simulink model "scattering_based_vel_vel"  (R2020b)
settings: Solver=ode45  StartTime=0.0  StopTime=10  RelTol=1e-3
values from neighbouring files (symbols this model uses):
  A = [1 Ts ... (first row only)    [kalman_hw6_main_vv.m]
  Amp = 0.8    [hw6_main_vv.m]    (also in kalman_hw6_main_vv.m = 0.3)
  b = 1    [hw6_main_vv.m]    (also in kalman_hw6_main_vv.m)
  Be = 20    [hw6_main_vv.m]    (also in kalman_hw6_main_vv.m)
  Bh = 1.5    [hw6_main_vv.m]    (also in kalman_hw6_main_vv.m)
  Bm = 10    [hw6_main_vv.m]    (also in kalman_hw6_main_vv.m)
  Bs = 100    [hw6_main_vv.m]    (also in kalman_hw6_main_vv.m)
  C = [1 0]    [kalman_hw6_main_vv.m]
  delay = 10    [hw6_main_vv.m]    (also in kalman_hw6_main_vv.m)
  Dh = 8    [hw6_main_vv.m]    (also in kalman_hw6_main_vv.m)
  Dm = 0    [hw6_main_vv.m]    (also in kalman_hw6_main_vv.m)
  Ds = 0    [hw6_main_vv.m]    (also in kalman_hw6_main_vv.m)
  Je = 0    [hw6_main_vv.m]    (also in kalman_hw6_main_vv.m)
  Jh = 0    [hw6_main_vv.m]    (also in kalman_hw6_main_vv.m)
  Ke = 210    [hw6_main_vv.m]    (also in kalman_hw6_main_vv.m)
  Kh = 0.1    [hw6_main_vv.m]    (also in kalman_hw6_main_vv.m)
  Km = 30    [hw6_main_vv.m]    (also in kalman_hw6_main_vv.m)
  Ks = 80    [hw6_main_vv.m]    (also in kalman_hw6_main_vv.m)
  Mm = 0.5    [hw6_main_vv.m]    (also in kalman_hw6_main_vv.m)
  Ms = 2    [hw6_main_vv.m]    (also in kalman_hw6_main_vv.m)
  Ph = 1    [hw6_main_vv.m]    (also in kalman_hw6_main_vv.m)
  posNoiseVar = 0.00001    (= 1e-05)    [kalman_hw6_main_vv.m]
  R_m = 1    [kalman_hw6_main_vv.m]
  R_s = 1    [kalman_hw6_main_vv.m]
  torqueNoiseVar = 0.01    [kalman_hw6_main_vv.m]
  Ts = 0.001    [hw6_main_vv.m]    (also in kalman_hw6_main_vv.m)
  xe = 0.5    [hw6_main_vv.m]    (also in kalman_hw6_main_vv.m)
undefined symbols (not defined in the file or in its folder): DiscIntNeverNeededParam, Discrete, Fc, Fip, Time
libraries: simulink x4, ctrlSharedLib x2
settings Model: Creator=nicol  LastModifiedBy=nicol

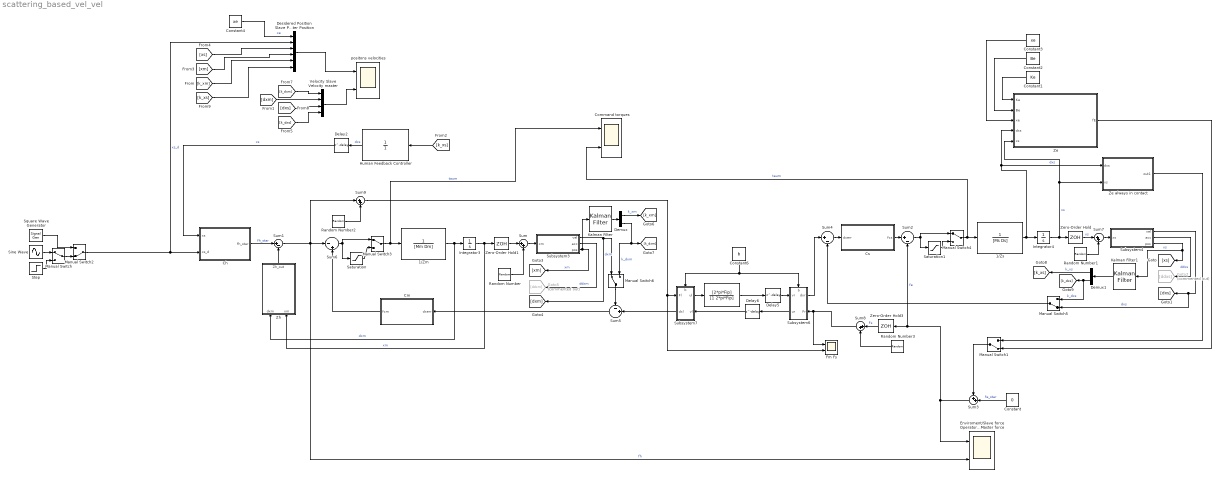
== system scattering_based_vel_vel ==
  " " : TransferFcn  Numerator=[2*pi*Fip]  Denominator=[1 2*pi*Fip]
  1/Zm : TransferFcn  Denominator=[Mm Dm]
  1/Zs : TransferFcn  Denominator=[Ms Ds]
  Ch : Subsystem
  Cm : Subsystem
  Command torques : Scope  NumInputPorts=2
  Constant : Constant  Value=0
  Constant1 : Constant  Value=Ke
  Constant2 : Constant  Value=Be
  Constant3 : Constant  Value=xe
  Constant4 : Constant  Value=xe
  Constant6 : Constant  Value=b
  Cs : Subsystem
  Delay2 : Delay  DelayLength=delay  SampleTime=Ts
  Delay5 : Delay  DelayLength=delay  SampleTime=Ts
  Delay6 : Delay  DelayLength=delay  SampleTime=Ts
  Demux : Demux  Outputs=2
  Demux1 : Demux  Outputs=2
  Desidered Position Slave Position Master Position : Mux  Inputs=6
  Enviroment/Slave force Operator/Master force : Scope  NumInputPorts=2
  Fm Fs : Scope  NumInputPorts=2
  Goto2 : Goto  Commented=on  GotoTag=ddxs
  Goto5 : Goto  Commented=on  GotoTag=ddxm
  Human Feedback Controller : TransferFcn  Denominator=[1]
  Integrator3 : Integrator
  Integrator4 : Integrator
  Kalman Filter : ctrlSharedLib/Kalman Filter  TimeDomain=Discrete-Time  UseCurrentEstimator=on  ModelSource=Individual A, B, C, D matrices  ModelSourceVariable=ss(0.95,1,0,0,Ts)  A=A  B=1  C=C  D=0  NumberOfStates=1  NumberOfInputs=1  NumberOfOutputs=1  InitialEstimateSource=Dialog  X0=0  P0=10  UseK=off  UseGH=off  NumberOfProcessNoiseInputs=1  G=1  TimeInvariantG=on  H=0  TimeInvariantH=on  Q=Q_m  TimeInvariantQ=on  R=R_m  TimeInvariantR=on  N=0  TimeInvariantN=on  AddInputPort=off  AddEnablePort=off  OutputEstimatedY=off  OutputP=off  Ts=Ts
  Kalman Filter1 : ctrlSharedLib/Kalman Filter  TimeDomain=Discrete-Time  UseCurrentEstimator=on  ModelSource=Individual A, B, C, D matrices  ModelSourceVariable=ss(0.95,1,0,0,Ts)  A=A  B=1  C=C  D=0  NumberOfStates=1  NumberOfInputs=1  NumberOfOutputs=1  InitialEstimateSource=Dialog  X0=0  P0=10  UseK=off  UseGH=off  NumberOfProcessNoiseInputs=1  G=1  TimeInvariantG=on  H=0  TimeInvariantH=on  Q=Q_s  TimeInvariantQ=on  R=R_s  TimeInvariantR=on  N=0  TimeInvariantN=on  AddInputPort=off  AddEnablePort=off  OutputEstimatedY=off  OutputP=off  Ts=Ts
  Manual Switch{,3..4,6} (4 alike) : ManualSwitch
  Manual Switch1 : ManualSwitch  CurrentSetting=0
  Manual Switch2 : ManualSwitch  CurrentSetting=0
  Manual Switch5 : ManualSwitch  CurrentSetting=0
  Random Number : RandomNumber  Variance=posNoiseVar  SampleTime=Ts
  Random Number1 : RandomNumber  Variance=posNoiseVar  SampleTime=Ts
  Random Number2 : RandomNumber  Variance=torqueNoiseVar  SampleTime=Ts
  Random Number3 : RandomNumber  Variance=torqueNoiseVar  SampleTime=Ts
  Saturation : Saturate  UpperLimit=50  LowerLimit=-50
  Saturation1 : Saturate  UpperLimit=50  LowerLimit=-50
  Sine Wave : Sin  Amplitude=Amp  Frequency=2*pi*Fc  SampleTime=0
  Square Wave Generator : SignalGenerator  WaveForm=square  Amplitude=Amp  Frequency=Fc  Units=rad/sec
  Step : Step  Time=Amp  SampleTime=0
  Subsystem3 : Subsystem
  Subsystem4 : Subsystem
  Subsystem6 : Subsystem
      settings: PortSchema="{\"entries\":[{\"content\":{\"sides\":[{\"content\":{\"connectorIds\":[\"In1\",\"Out2\"]},\"type\":\"ConnectorPlacement.EquallySpacedRectSide\",\"uuid\":\"6288401b-7cd3-4b91-bca2-5e472b2e7daa\"},{\"content\":{\"connectorIds\":[\"Out1\",\"In3\"],\"side\":\"RIGHT\"},\"type\":\"ConnectorPlacement.EquallySpacedRectSide\",\"uuid\":\"a26b0e98-9a48-48c5-be40-0718b6388037\"},{\"content\":{\"connectorIds\":[\"In2\"],\"side\":\"TOP\"},\"type\":\"ConnectorPlacement.EquallySpacedRectSide\",\"uuid\":\"663684a5-b6d6-4ce8-bd22-863e832b1e44\"},{\"content\":{\"connectorIds\":[],\"side\":\"HIDDEN\"},\"type\":\"ConnectorPlacement.EquallySpacedRectSide\",\"uuid\":\"305185ea-b8ab-4d44-85aa-b4ee32720aa4\"}]},\"type\":\"ConnectorPlacement.EquallySpacedConnector\",\"uuid\":\"5d1994be-23eb-41de-9d91-33fb6a380aab\"}],\"packageUris\":[\"http://schema.mathworks.com/mf0/Connector/R2020b\"],\"version\":\"1.0\"}"
  Subsystem7 : Subsystem
      settings: PortSchema="{\"entries\":[{\"content\":{\"sides\":[{\"content\":{\"connectorIds\":[\"In1\",\"Out2\"]},\"type\":\"ConnectorPlacement.EquallySpacedRectSide\",\"uuid\":\"6288401b-7cd3-4b91-bca2-5e472b2e7daa\"},{\"content\":{\"connectorIds\":[\"Out1\",\"In3\"],\"side\":\"RIGHT\"},\"type\":\"ConnectorPlacement.EquallySpacedRectSide\",\"uuid\":\"a26b0e98-9a48-48c5-be40-0718b6388037\"},{\"content\":{\"connectorIds\":[\"In2\"],\"side\":\"TOP\"},\"type\":\"ConnectorPlacement.EquallySpacedRectSide\",\"uuid\":\"663684a5-b6d6-4ce8-bd22-863e832b1e44\"},{\"content\":{\"connectorIds\":[],\"side\":\"HIDDEN\"},\"type\":\"ConnectorPlacement.EquallySpacedRectSide\",\"uuid\":\"305185ea-b8ab-4d44-85aa-b4ee32720aa4\"}]},\"type\":\"ConnectorPlacement.EquallySpacedConnector\",\"uuid\":\"5d1994be-23eb-41de-9d91-33fb6a380aab\"}],\"packageUris\":[\"http://schema.mathworks.com/mf0/Connector/R2020b\"],\"version\":\"1.0\"}"
  Sum{,7..9} (4 alike) : Sum  Inputs=|++
  Sum1 : Sum  Inputs=|+-
  Sum2 : Sum  Inputs=|+-
  Sum3 : Sum  Inputs=++|
  Sum4 : Sum  Inputs=|+-
  Sum5 : Sum  Inputs=-+|
  Sum6 : Sum  Inputs=|-+
  Velocity Slave Velocity master : Mux
  Ze : MATLAB Function  TreatAsAtomicUnit=on
  Ze always in contact : Subsystem
  Zero-Order Hold : ZeroOrderHold  SampleTime=Ts
  Zero-Order Hold1 : ZeroOrderHold  SampleTime=Ts
  Zero-Order Hold3 : ZeroOrderHold  SampleTime=Ts
  Zh : Subsystem
  "positons velocities " : Scope  NumInputPorts=2
  wires:
  Ch/1(fh_star) -> Sum1/1  "fh_star"
  Zh/1(Zh_out) -> Sum1/2
  1/Zm/1 -> Integrator3/1, Zh/1(dxm)  "dxm"
  Sum1/1 -> Sum9/1, Sum6/1, Enviroment/Slave force Operator/Master force/2  "fh"
  Cs/1(fcs) -> Sum2/1
  1/Zs/1 -> Integrator4/1, Ze always in contact/1(dxs), Ze/4(dxs)  "dxs"
  Ze/1(fE) -> Manual Switch1/2
  Sum3/1 -> Enviroment/Slave force Operator/Master force/1, Zero-Order Hold3/1, Sum2/2  "fe"
  Constant/1 -> Sum3/2  "fe_star"
  Constant1/1 -> Ze/1(Ke)
  Constant2/1 -> Ze/2(Be)
  Constant3/1 -> Ze/3(xe)
  Integrator4/1 -> Zero-Order Hold/1, Ze/5(xs), Ze always in contact/2(xs)  "xs"
  Sine Wave/1 -> Manual Switch/1
  Manual Switch1/1 -> Sum3/1
  Ze always in contact/1(out1) -> Manual Switch1/1
  Sum4/1 -> Cs/1(dxerr)
  Subsystem3/1(vel) -> Manual Switch6/1, [dxm]  "dxm"
  Subsystem3/3(pos) -> Kalman Filter/1, [xm]  "xm"
  Integrator3/1 -> Zero-Order Hold1/1, Zh/2(xm)  "xm"
  Subsystem3/2(acc) -> Goto5/1  "ddxm"
  Zero-Order Hold1/1 -> Sum/1
  Subsystem4/2(acc) -> Goto2/1  "ddxs"
  Subsystem4/1(vel) -> Manual Switch5/2, [dxs]  "dxs"
  Subsystem4/3(pos) -> Kalman Filter1/1, [xs]  "xs"
  Zero-Order Hold/1 -> Sum7/1  "xs"
  [k_xs] -> Human Feedback Controller/1
  Subsystem6/1(dxr) -> Sum4/1
  Zero-Order Hold3/1 -> Sum8/1  "Fs"
  Subsystem7/1(ul) -> " "/1
  Delay5/1 -> Subsystem6/1(vr)
  Subsystem6/2(ur) -> Delay6/1
  Constant6/1 -> Subsystem7/2(b), Subsystem6/2(b)
  " "/1 -> Delay5/1
  Subsystem7/2(dxl) -> Sum5/2
  Delay6/1 -> Subsystem7/3(vl)
  Cm/1(fcm) -> Sum6/2
  Sum5/1 -> Cm/1(dxerr)
  Square Wave Generator/1 -> Manual Switch2/1
  Kalman Filter/1 -> Demux/1
  Demux/2 -> [k_dxm], Manual Switch6/2  "k_dxm"
  Demux/1 -> [k_xm]  "k_xm"
  Demux1/1 -> [k_xs]  "k_xs"
  Kalman Filter1/1 -> Demux1/1
  Demux1/2 -> Manual Switch5/1, [k_dxs]  "k_dxs"
  Constant4/1 -> Desidered Position Slave Position Master Position/1  "xe"
  Manual Switch2/1 -> Desidered Position Slave Position Master Position/2, Ch/2(xs_d)  "xs_d"
  [k_dxm] -> Velocity Slave Velocity master/1
  [dxs] -> Velocity Slave Velocity master/3
  Human Feedback Controller/1 -> Delay2/1  "dxs"
  Velocity Slave Velocity master/1 -> "positons velocities "/2
  [xs] -> Desidered Position Slave Position Master Position/3
  Delay2/1 -> Ch/1(xs)  "xs"
  [dxm] -> Velocity Slave Velocity master/2
  Desidered Position Slave Position Master Position/1 -> "positons velocities "/1
  Sum/1 -> Subsystem3/1(xm)
  Random Number/1 -> Sum/2
  Sum7/1 -> Subsystem4/1(xs)
  Random Number1/1 -> Sum7/2
  Random Number3/1 -> Sum8/2
  Sum8/1 -> Fm Fs/1, Subsystem6/3(Fr)
  Sum9/1 -> Subsystem7/1(Fl), Fm Fs/2
  Random Number2/1 -> Sum9/2
  Manual Switch/1 -> Manual Switch2/2
  Step/1 -> Manual Switch/2
  [xm] -> Desidered Position Slave Position Master Position/4
  [k_xm] -> Desidered Position Slave Position Master Position/5
  [k_xs] -> Desidered Position Slave Position Master Position/6
  Manual Switch3/1 -> Command torques/1, 1/Zm/1  "taum"
  Sum6/1 -> Manual Switch3/1, Saturation/1
  Saturation/1 -> Manual Switch3/2
  Sum2/1 -> Manual Switch4/1, Saturation1/1
  Saturation1/1 -> Manual Switch4/2
  Manual Switch4/1 -> Command torques/2, 1/Zs/1  "taum"
  [k_dxs] -> Velocity Slave Velocity master/4
  Manual Switch5/1 -> Sum4/2
  Manual Switch6/1 -> Sum5/1

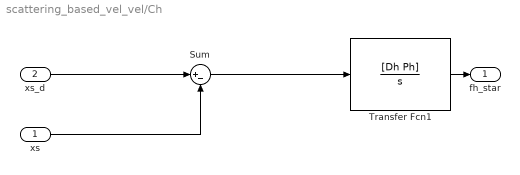
== system scattering_based_vel_vel/Ch ==
  xs : Inport
  xs_d : Inport  Port=2
  Sum : Sum  Inputs=|+-
  Transfer Fcn1 : TransferFcn  Numerator=[Dh Ph]  Denominator=[1 0]
  fh_star : Outport
  wires:
  xs/1 -> Sum/2
  Sum/1 -> Transfer Fcn1/1
  Transfer Fcn1/1 -> fh_star/1
  xs_d/1 -> Sum/1

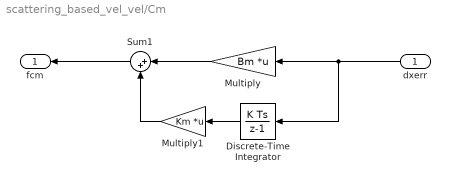
== system scattering_based_vel_vel/Cm ==
  dxerr : Inport
  Discrete-Time Integrator : DiscreteIntegrator  SampleTime=-1  ICPrevOutput=DiscIntNeverNeededParam  ICPrevScaledInput=DiscIntNeverNeededParam
  Multiply : Gain  Gain=Bm  Multiplication=Matrix(K*u)
  Multiply1 : Gain  Gain=Km  Multiplication=Matrix(K*u)
  Sum1 : Sum  Inputs=|++
  fcm : Outport
  wires:
  dxerr/1 -> Discrete-Time Integrator/1, Multiply/1
  Multiply1/1 -> Sum1/2
  Multiply/1 -> Sum1/1
  Sum1/1 -> fcm/1
  Discrete-Time Integrator/1 -> Multiply1/1

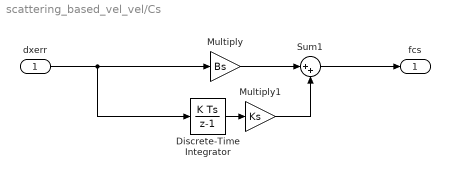
== system scattering_based_vel_vel/Cs ==
  dxerr : Inport
  Discrete-Time Integrator : DiscreteIntegrator  SampleTime=-1  ICPrevOutput=DiscIntNeverNeededParam  ICPrevScaledInput=DiscIntNeverNeededParam
  Multiply : Gain  Gain=Bs
  Multiply1 : Gain  Gain=Ks
  Sum1 : Sum  Inputs=|++
  fcs : Outport
  wires:
  dxerr/1 -> Discrete-Time Integrator/1, Multiply/1
  Multiply1/1 -> Sum1/2
  Multiply/1 -> Sum1/1
  Sum1/1 -> fcs/1
  Discrete-Time Integrator/1 -> Multiply1/1

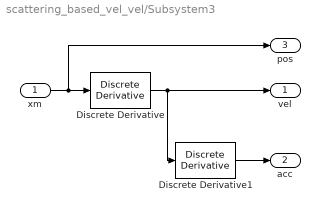
== system scattering_based_vel_vel/Subsystem3 ==
  xm : Inport
  Discrete Derivative : simulink/Discrete/Discrete Derivative  gainval=1.0  ICPrevScaledInput=0.0  OutMin=[]  OutMax=[]  OutDataType=fixdt(1, 16)  OutScaling=2^-10  DoSatur=off
  Discrete Derivative1 : simulink/Discrete/Discrete Derivative  gainval=1.0  ICPrevScaledInput=0.0  OutMin=[]  OutMax=[]  OutDataType=fixdt(1, 16)  OutScaling=2^-10  DoSatur=off
  vel : Outport
  acc : Outport  Port=2
  pos : Outport  Port=3
  wires:
  xm/1 -> pos/1, Discrete Derivative/1
  Discrete Derivative/1 -> Discrete Derivative1/1, vel/1
  Discrete Derivative1/1 -> acc/1

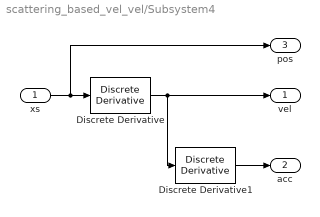
== system scattering_based_vel_vel/Subsystem4 ==
  xs : Inport
  Discrete Derivative : simulink/Discrete/Discrete Derivative  gainval=1.0  ICPrevScaledInput=0.0  OutMin=[]  OutMax=[]  OutDataType=fixdt(1, 16)  OutScaling=2^-10  DoSatur=off
  Discrete Derivative1 : simulink/Discrete/Discrete Derivative  gainval=1.0  ICPrevScaledInput=0.0  OutMin=[]  OutMax=[]  OutDataType=fixdt(1, 16)  OutScaling=2^-10  DoSatur=off
  vel : Outport
  acc : Outport  Port=2
  pos : Outport  Port=3
  wires:
  xs/1 -> pos/1, Discrete Derivative/1
  Discrete Derivative/1 -> Discrete Derivative1/1, vel/1
  Discrete Derivative1/1 -> acc/1

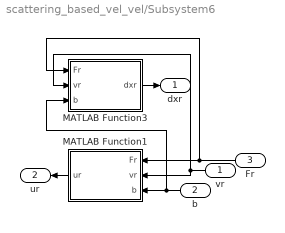
== system scattering_based_vel_vel/Subsystem6 ==
  vr : Inport
  b : Inport  Port=2
  Fr : Inport  Port=3
  MATLAB Function1 : MATLAB Function  TreatAsAtomicUnit=on
  MATLAB Function3 : MATLAB Function  TreatAsAtomicUnit=on
  dxr : Outport
  ur : Outport  Port=2
  wires:
  MATLAB Function1/1(ur) -> ur/1
  MATLAB Function3/1(dxr) -> dxr/1
  vr/1 -> MATLAB Function1/2(vr), MATLAB Function3/2(vr)
  Fr/1 -> MATLAB Function3/1(Fr), MATLAB Function1/1(Fr)
  b/1 -> MATLAB Function3/3(b), MATLAB Function1/3(b)

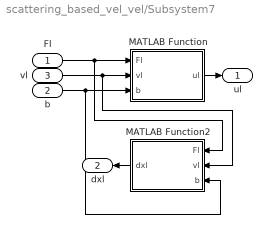
== system scattering_based_vel_vel/Subsystem7 ==
  Fl : Inport
  b : Inport  Port=2
  vl : Inport  Port=3
  MATLAB Function : MATLAB Function  TreatAsAtomicUnit=on
  MATLAB Function2 : MATLAB Function  TreatAsAtomicUnit=on
  ul : Outport
  dxl : Outport  Port=2
  wires:
  b/1 -> MATLAB Function2/3(b), MATLAB Function/3(b)
  vl/1 -> MATLAB Function2/2(vl), MATLAB Function/2(vl)
  Fl/1 -> MATLAB Function2/1(Fl), MATLAB Function/1(Fl)
  MATLAB Function2/1(dxl) -> dxl/1
  MATLAB Function/1(ul) -> ul/1

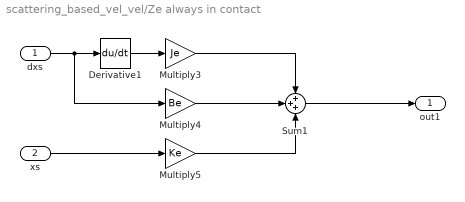
== system scattering_based_vel_vel/Ze always in contact ==
  dxs : Inport
  xs : Inport  Port=2
  Derivative1 : Derivative
  Multiply3 : Gain  Gain=Je
  Multiply4 : Gain  Gain=Be
  Multiply5 : Gain  Gain=Ke
  Sum1 : Sum  Inputs=+++
  out1 : Outport
  wires:
  Sum1/1 -> out1/1
  Multiply4/1 -> Sum1/2
  Multiply5/1 -> Sum1/3
  dxs/1 -> Multiply4/1, Derivative1/1
  Derivative1/1 -> Multiply3/1
  xs/1 -> Multiply5/1
  Multiply3/1 -> Sum1/1

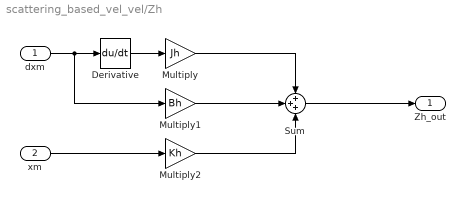
== system scattering_based_vel_vel/Zh ==
  dxm : Inport
  xm : Inport  Port=2
  Derivative : Derivative
  Multiply : Gain  Gain=Jh
  Multiply1 : Gain  Gain=Bh
  Multiply2 : Gain  Gain=Kh
  Sum : Sum  Inputs=+++
  Zh_out : Outport
  wires:
  dxm/1 -> Multiply1/1, Derivative/1
  Derivative/1 -> Multiply/1
  Sum/1 -> Zh_out/1
  xm/1 -> Multiply2/1
  Multiply1/1 -> Sum/2
  Multiply/1 -> Sum/1
  Multiply2/1 -> Sum/3

== matlab function scattering_based_vel_vel/Ze ==
  data: Ke input; fE output; Be input; xe input; dxs input; xs input
function fE = environment(Ke,Be,xe,dxs,xs)
if(xs>xe)
    fE=Ke*(xs-xe)+Be*dxs;
else
    fE=0;
end

== matlab function scattering_based_vel_vel/Subsystem7/MATLAB Function ==
  data: Fl input; ul output; vl input; b input
function ul = fcn(Fl,vl,b)
ul = sqrt(2/b)*Fl-vl;

== matlab function scattering_based_vel_vel/Subsystem6/MATLAB Function1 ==
  data: Fr input; ur output; vr input; b input
function ur = fcn(Fr,vr,b)
ur = sqrt(2/b)*Fr-vr;

== matlab function scattering_based_vel_vel/Subsystem7/MATLAB Function2 ==
  data: Fl input; dxl output; vl input; b input
function dxl = fcn(Fl,vl,b)
dxl = (Fl-sqrt(2*b)*vl)/b;

== matlab function scattering_based_vel_vel/Subsystem6/MATLAB Function3 ==
  data: Fr input; dxr output; vr input; b input
function dxr = fcn(Fr,vr,b)
dxr = -(Fr-sqrt(2*b)*vr)/b;
